simulink model "verify_THB_set_T_mdl"  (R2016b)
settings: Solver=VariableStepDiscrete  StartTime=0  StopTime=10  MaxStep=1  RelTol=1e-3  EnableMultiTasking=on
InitFcn:
  | load('DE_TRY2010_13_averageYear')
libraries: carnot x2, simulink x1
settings Model: Creator=drhf  LastModifiedBy=User
settings DataIOCC: SaveFormat=Array  SignalLoggingSaveFormat=ModelDataLogs
settings OptimizationCC: ExpressionDepthLimit=2147483647  LifeSpan=inf
settings DebuggingCC: UnderspecifiedInitializationDetection=Classic  MergeDetectMultiDrivingBlocksExec=none  SolverPrmCheckMsg=warning  FcnCallInpInsideContextMsg=warning  StateNameClashWarn=warning  SFUnexpectedBacktrackingDiag=warning  SFNoUnconditionalDefaultTransitionDiag=warning  SFExecutionAtInitializationDiag=none
settings HardwareCC: ProdBitPerPointer=32  ProdBitPerSizeT=32  ProdBitPerPtrDiffT=32  ProdLargestAtomicFloat=None  ProdIntDivRoundTo=Undefined  ProdEndianess=Unspecified  ProdWordSize=32  ProdHWDeviceType=32-bit Generic
settings ModelReferenceCC: PropagateSignalLabelsOutOfModel=off
settings GRTTargetCC: TargetLangStandard=C89/C90 (ANSI)  GeneratePreprocessorConditionals=Disable all  CombineOutputUpdateFcns=off  GRTInterface=on
settings ConfigComp: CovMetricSettings=dw  CovHtmlReporting=on  CovSaveCumulativeToWorkspaceVar=on  CovSaveSingleToWorkspaceVar=on  CovExternalEMLEnable=off

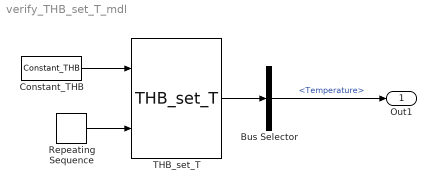
== system verify_THB_set_T_mdl ==
  Bus Selector : BusSelector  OutputSignals=Temperature
  Constant_THB : carnot/Source/Simple/Constant_THB  t=20  mdot=0  p=1e5  mID=No Pressure Drop  fluid=Water  mix=0  mix2=0  mix3=0  dia=0.02  hgt=0
  Repeating Sequence : simulink/Sources/Repeating Sequence  rep_seq_t=[0 5 10]  rep_seq_y=[30 60 30]
  THB_set_T : carnot/Source/Simple/THB_set_T
  Out1 : Outport
  wires:
  THB_set_T/1 -> Bus Selector/1
  Bus Selector/1 -> Out1/1  "<Temperature>"
  Constant_THB/1 -> THB_set_T/1
  Repeating Sequence/1 -> THB_set_T/2
